simulink model "Simulation_1_model"  (R2017b)
settings: Solver=ode23tb  StartTime=0.0  StopTime=.05  MaxStep=1e-6  RelTol=1e-3
values from neighbouring files (symbols this model uses):
  d = Va/Vdc    (= 0.403199081699)    [Simulation_1_code.m]    (also in Simulation_2_code.m)
  ea = ke*w    (= 78.5398163397)    [Simulation_1_code.m]    (also in Simulation_2_code.m)
  fs = 25000    [Simulation_1_code.m]    (also in Simulation_2_code.m)
  La = 1.5e-3    (= 0.0015)    [Simulation_1_code.m]    (also in Simulation_2_code.m)
  Ra = 0.35    [Simulation_1_code.m]    (also in Simulation_2_code.m)
  Vdc = 200    [Simulation_1_code.m]    (also in Simulation_2_code.m)
libraries: powerlib x10, simulink x1
settings Model: Creator=Jess  LastModifiedBy=Andrew McCullough

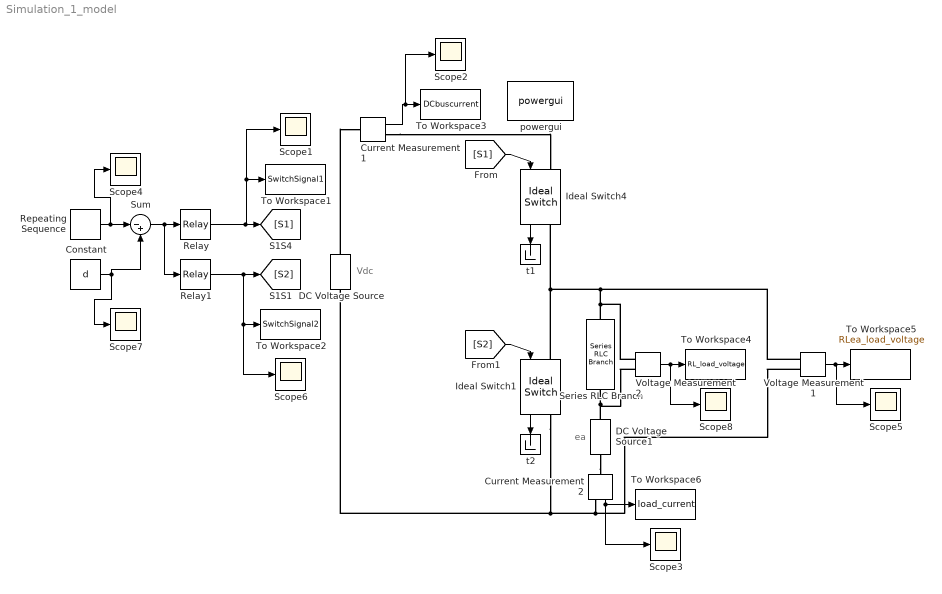
== system Simulation_1_model ==
  note: ea
  note: Vdc
  Constant : Constant  Value=d
  Current Measurement1 : powerlib/Measurements/Current Measurement  PhasorSimulation=off  OutputType=Complex  PSBequivalent=0
  Current Measurement2 : powerlib/Measurements/Current Measurement  PhasorSimulation=off  OutputType=Complex  PSBequivalent=0
  DC Voltage Source : powerlib/Electrical Sources/DC Voltage Source  Amplitude=Vdc  Measurements=None
  DC Voltage Source1 : powerlib/Electrical Sources/DC Voltage Source  Amplitude=ea  Measurements=None
  Ideal Switch1 : powerlib/Power Electronics/Ideal Switch  Ron=0.001  Lon=0  IC=0  Rs=1e5  Cs=inf  Measurements=on
  Ideal Switch4 : powerlib/Power Electronics/Ideal Switch  Ron=0.001  Lon=0  IC=0  Rs=1e5  Cs=inf  Measurements=on
  Relay : Relay
  Relay1 : Relay  OnOutputValue=0  OffOutputValue=1
  Repeating Sequence : simulink/Sources/Repeating Sequence  rep_seq_t=[0 0.5/fs 1/fs]  rep_seq_y=[0 1 0]
  Scope{1..8} (8 alike) : Scope
  Series RLC Branch : powerlib/Elements/Series RLC Branch  LConnTagsString=__new0  RConnTagsString=__new0  BranchType=RL  Resistance=Ra  Inductance=La  SetiL0=off  InitialCurrent=0  Capacitance=inf  Setx0=off  InitialVoltage=0  Measurements=None
  Sum : Sum  Inputs=|-+
  To Workspace1 : ToWorkspace  VariableName=SwitchSignal1  SaveFormat=Timeseries  SampleTime=-1
  To Workspace2 : ToWorkspace  VariableName=SwitchSignal2  SaveFormat=Timeseries  SampleTime=-1
  To Workspace3 : ToWorkspace  VariableName=DCbuscurrent  SaveFormat=Structure With Time  SampleTime=-1
  To Workspace4 : ToWorkspace  VariableName=RL_load_voltage  SaveFormat=Timeseries  SampleTime=-1
  To Workspace5 : ToWorkspace  VariableName=RLea_load_voltage  SaveFormat=Timeseries  SampleTime=-1
  To Workspace6 : ToWorkspace  VariableName=load_current  SaveFormat=Timeseries  SampleTime=-1
  Voltage Measurement1 : powerlib/Measurements/Voltage Measurement  PhasorSimulation=off  OutputType=Complex  PSBequivalent=0
  Voltage Measurement2 : powerlib/Measurements/Voltage Measurement  PhasorSimulation=off  OutputType=Complex  PSBequivalent=0
  powergui : powerlib/powergui  Priority=1  SimulationMode=Continuous  SampleTime=50e-6  frequency=60  Iterations=50  frequencyindice=0  Pbase=100e6  ErrMax=1e-4  UnitsV=kV  UnitsW=MW  buscounter=0  FunctionMessages=off  echomessages=off  EnableUseOfTLC=off  CurrentSourceSwitches=off  DisableSnubberDevices=off  DisableRonSwitches=off  DisableVfSwitches=off  DisplayEquations=off  SolverType=Tustin/Backward Euler (TBE)  Interpol=off  ExternalGateDelay=off  methode=off  Ts=100  x0status=blocks  SPID=on  SwTol=0  HookPort=off  RestoreLinks=warning  ResistiveCurrentMeasurement=off  Frange=[0:2:500]  Ylog=off  Xlog=on  ShowGrid=off  save=off  variable=ZData  structure=voltage  ZoomFFT=off  StartTime=0.0  cycles=10  DisplayStyle=1  fundamental=100  FreqAxis=off  MaxFrequency=1000  frequencyindicesteady=1  RmsSteady=1  display=off
  t1 : Terminator
  t2 : Terminator
  wires:
  [S1] -> Ideal Switch4/1
  Current Measurement1/1 -> Scope2/1, To Workspace3/1
  Relay/1 -> [S1], To Workspace1/1, Scope1/1
  [S2] -> Ideal Switch1/1
  Ideal Switch1/1 -> t2/1
  Ideal Switch4/1 -> t1/1
  Current Measurement2/1 -> To Workspace6/1, Scope3/1
  Repeating Sequence/1 -> Scope4/1, Sum/1
  Constant/1 -> Sum/2, Scope7/1
  Sum/1 -> Relay1/1, Relay/1
  Relay1/1 -> To Workspace2/1, Scope6/1, [S2]
  Voltage Measurement2/1 -> To Workspace4/1, Scope8/1
  Voltage Measurement1/1 -> Scope5/1, To Workspace5/1
  connections:
  DC Voltage Source/RConn1 -- Current Measurement1/LConn1
  Series RLC Branch/RConn1 -- Voltage Measurement2/LConn1 -- Voltage Measurement1/LConn1 -- Ideal Switch1/LConn1 -- Ideal Switch4/RConn1
  Voltage Measurement1/LConn2 -- Current Measurement2/RConn1 -- Ideal Switch1/RConn1 -- DC Voltage Source/LConn1
  Current Measurement1/RConn1 -- Ideal Switch4/LConn1
  DC Voltage Source1/LConn1 -- Current Measurement2/LConn1
  DC Voltage Source1/RConn1 -- Voltage Measurement2/LConn2 -- Series RLC Branch/LConn1
